simulink model "chap4_7sim"  (Simulink 3.00)
settings: Solver=ode45  StartTime=0.0  StopTime=20  RelTol=1e-3
settings Model: LastModifiedBy=liu

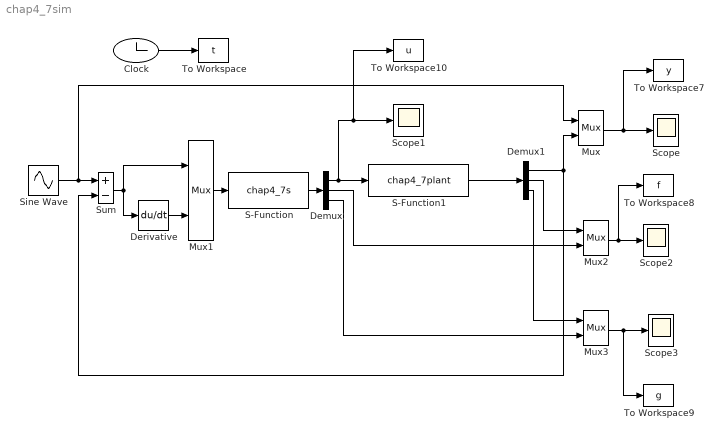
== system chap4_7sim ==
  Clock : Clock
  Demux : Demux  Outputs=3
  Demux1 : Demux  Outputs=3
  Derivative : Derivative
  Mux{,1..3} (4 alike) : Mux  Inputs=2
      settings: DisplayOption=none
  S-Function : S-Function  FunctionName=chap4_7s  PortCounts=[]  SFunctionModules=''
  S-Function1 : S-Function  FunctionName=chap4_7plant  PortCounts=[]  SFunctionModules=''
  Scope{,1..3} (4 alike) : Scope
      Scope settings: TimeRange=3  YMin=-0.11  YMax=0.1  SaveToWorkspace=off  SaveName=ScopeData  MaxRows=500000
      Scope1 settings: TimeRange=3  YMin=-1.75  YMax=1.75  SaveToWorkspace=off  SaveName=ScopeData  MaxRows=500000
      Scope2 settings: TimeRange=3  YMin=-0.1  YMax=1  SaveToWorkspace=off  SaveName=ScopeData  MaxRows=500000
      Scope3 settings: TimeRange=3  YMin=0  YMax=140  SaveToWorkspace=off  SaveName=ScopeData  MaxRows=500000
  Sine Wave : Sin  Amplitude=0.1  Frequency=1  Phase=0  SampleTime=0
  Sum : Sum  Inputs=+-  SaturateOnIntegerOverflow=on
  To Workspace : ToWorkspace  VariableName=t  SampleTime=-1  SaveFormat=Matrix
  To Workspace10 : ToWorkspace  VariableName=u  SampleTime=-1  SaveFormat=Matrix
  To Workspace7 : ToWorkspace  VariableName=y  SampleTime=-1  SaveFormat=Matrix
  To Workspace8 : ToWorkspace  VariableName=f  SampleTime=-1  SaveFormat=Matrix
  To Workspace9 : ToWorkspace  VariableName=g  SampleTime=-1  SaveFormat=Matrix
  wires:
  Mux1/1 -> S-Function/1
  S-Function/1 -> Demux/1
  Demux/1 -> S-Function1/1, Scope1/1, To Workspace10/1
  S-Function1/1 -> Demux1/1
  Derivative/1 -> Mux1/2
  Demux1/1 -> Sum/2, Mux/2
  Demux1/2 -> Mux2/1
  Demux1/3 -> Mux3/1
  Mux/1 -> Scope/1, To Workspace7/1
  Mux2/1 -> Scope2/1, To Workspace8/1
  Mux3/1 -> Scope3/1, To Workspace9/1
  Demux/2 -> Mux2/2
  Demux/3 -> Mux3/2
  Clock/1 -> To Workspace/1
  Sum/1 -> Mux1/1, Derivative/1
  Sine Wave/1 -> Sum/1, Mux/1
